simulink model "crane_sim"  (R2020a)
settings: Solver=FixedStepAuto  StartTime=0.0  StopTime=10  FixedStep=0.01  RelTol=1e-3
settings Model: Creator=controls  LastModifiedBy=controls

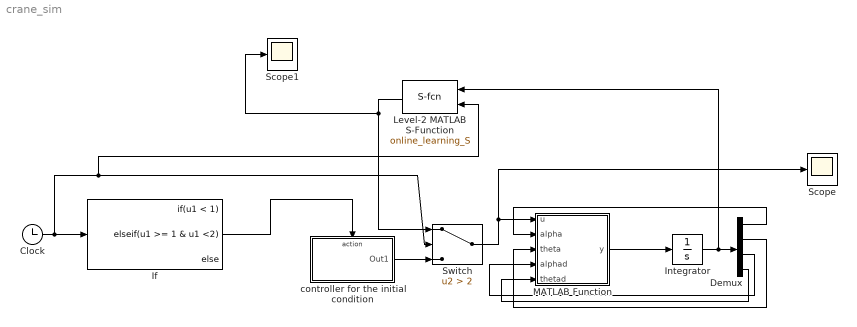
== system crane_sim ==
  Clock : Clock
  Demux : Demux
  If : If  IfExpression=u1 < 1  ElseIfExpressions=u1 >= 1 & u1 <2
  Integrator : Integrator
  Level-2 MATLAB S-Function : M-S-Function  FunctionName=online_learning_S
  MATLAB Function : MATLAB Function  TreatAsAtomicUnit=on
  Scope : Scope
  Scope1 : Scope
  Switch : Switch  Criteria=u2 > Threshold  Threshold=2
  controller for the initial condition : Subsystem  TreatAsAtomicUnit=on
  wires:
  MATLAB Function/1(y) -> Integrator/1
  If/2 -> controller for the initial condition/Action
  Clock/1 -> Level-2 MATLAB S-Function/2, Switch/2, If/1
  Integrator/1 -> Level-2 MATLAB S-Function/1, Demux/1
  Demux/1 -> MATLAB Function/2(alpha)
  Demux/2 -> MATLAB Function/3(theta)
  Demux/3 -> MATLAB Function/4(alphad)
  Demux/4 -> MATLAB Function/5(thetad)
  Switch/1 -> Scope/1, MATLAB Function/1(u)
  controller for the initial condition/1(Out1) -> Switch/3
  Level-2 MATLAB S-Function/1 -> Switch/1, Scope1/1

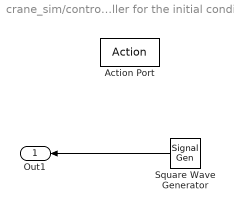
== system crane_sim/controller for the initial condition ==
  Action Port : ActionPort  ActionPortLabel=elseif(u1 >= 1 & u1 <2)
  Square Wave Generator : SignalGenerator  WaveForm=square
  Out1 : Outport
  wires:
  Square Wave Generator/1 -> Out1/1

== matlab function crane_sim/MATLAB Function ==
  data: u input; alpha input; y output; theta input; alphad input; thetad input
function y = fcn(u,alpha,theta,alphad,thetad)
 
    m = 0.114;
    J = 0.0076;
    l = 0.337;
    r = 0.216;
    g = 9.81;
    K1 = 0.2065;
    K2 = 0.1105;


    alpha_dot = alphad;
    theta_dot = thetad;

    tau = K1*u - K2*alpha_dot;

    denom = J + m*r^2 + m*l^2*sin(theta)^2-m*r^2*cos(theta)^2;
    alpha_ddot = (tau-m*r*l*cos(theta)*(alphad^2*sin(theta)*cos(theta)-g*sin(theta)/l)+m*r*l*thetad^2*sin(theta) - 2*m*l^2*alphad*thetad*sin(theta)*cos(theta)) / denom;

    K = J + m*r^2+m*l^2*sin(theta)^2;
    thetaddot_numer = -(r/l)*(tau + m*r*l*thetad^2*sin(theta)-2*m*l^2*alphad*thetad*sin(theta)*cos(theta))*cos(theta)/K + alphad^2*sin(theta)*cos(theta)-g*sin(theta)/l;
    thetaddot_denom = 1 - m*r^2*cos(theta)^2/K;
    theta_ddot = thetaddot_numer/thetaddot_denom;
    f = [alpha_dot;theta_dot;alpha_ddot;theta_ddot];
y = f;
